simulink model "ch6q1"  (R2019a)
settings: Solver=VariableStepAuto  StartTime=0.0  StopTime=8.0  RelTol=1e-3
settings Model: Creator=Administrator  LastModifiedBy=Administrator
settings OptimizationCC: BooleanDataType=off

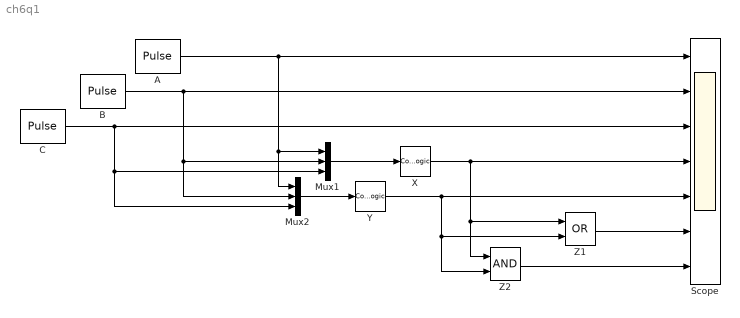
== system ch6q1 ==
  A : DiscretePulseGenerator  PhaseDelay=1  SampleTime=4
  B : DiscretePulseGenerator  PhaseDelay=1  SampleTime=2  VectorParams1D=off
  "C " : DiscretePulseGenerator  PhaseDelay=1
  Mux1 : Mux  Inputs=3
  Mux2 : Mux  Inputs=3
  Scope : Scope  NumInputPorts=7
  X : CombinatorialLogic  TruthTable=[1;1;1;1;1;1;1;0]
  Y : CombinatorialLogic  TruthTable=[1;0;0;0;0;0;0;1]
  Z1 : Logic  Operator=OR  AllPortsSameDT=off  OutDataTypeStr=boolean
  Z2 : Logic  AllPortsSameDT=off  OutDataTypeStr=boolean
  wires:
  B/1 -> Mux2/2, Mux1/2, Scope/2
  "C "/1 -> Mux1/3, Mux2/3, Scope/3
  Mux1/1 -> X/1
  A/1 -> Mux2/1, Mux1/1, Scope/1
  X/1 -> Z2/1, Z1/1, Scope/4
  Y/1 -> Z2/2, Z1/2, Scope/5
  Z1/1 -> Scope/6
  Z2/1 -> Scope/7
  Mux2/1 -> Y/1
